simulink model "DYNctl_ver4_etud_Avec_AsservissementNONfonctionnel"  (R2021b)
settings: Solver=ode45  StartTime=0.0  StopTime=tfin  FixedStep=0.001  RelTol=1e-09  EnableMultiTasking=on
values from neighbouring files (symbols this model uses):
  A = num_pos_sph(3)    [Compensateur.m]    (also in matrice_L.m = sym(zeros(13, 13)))
  ae0 = 0.000013398315537 * 1.0e+5    (= 1.3398315537)    [bancEssaiConstantes.m]
  ae1 = 0.003556457401249 * 1.0e+5    (= 355.645740125)    [bancEssaiConstantes.m]
  ae2 = 0.018168930792891 * 1.0e+5    (= 1816.89307929)    [bancEssaiConstantes.m]
  ae3 = 7.043847497815494 * 1.0e+5    (= 704384.749782)    [bancEssaiConstantes.m]
  as0 = 0.0609    [bancEssaiConstantes.m]
  as1 = 18.1233    [bancEssaiConstantes.m]
  as2 = 3.1142e+03    (= 3114.2)    [bancEssaiConstantes.m]
  as3 = -2.3281e+05    (= -232810)    [bancEssaiConstantes.m]
  Axeq = 0    [run_bancessai.m]
  Ayeq = 0    [run_bancessai.m]
  B = [B1 ... (first row only)    [matrice_L.m]
  be1 = 13.029359254409743    (= 13.0293592544)    [bancEssaiConstantes.m]
  C = [Tdef C3 C3 C3 C2 ... (first row only)    [matrice_L.m]
  D = [sum(distance);sum(distance.*voltage)]    [Capteur.m]    (also in matrice_L.m = [0])
  g = 9.81    [bancEssaiConstantes.m]    (also in courant_voltage.m; matrice_L.m; projet.m; trajectoire.m = sqrt(1+(yd).^2))
  Jy = Jx    (= 0.001169)    [bancEssaiConstantes.m]    (also in courant_voltage.m = 0.001347; matrice_L.m = 0.001347)
  Kp_pos_sph = (wn_pos_sph^2)/A_pos_sph    [Compensateur_position_sphere.m]
  Kv_pos_sph = (2*zeta_pos_sph*wn_pos_sph)/A_pos_sph    [Compensateur_position_sphere.m]
  LA = LL    (= 0.115)    [bancEssaiConstantes.m]
  LB = LL    (= 0.115)    [bancEssaiConstantes.m]
  LC = LL    (= 0.115)    [bancEssaiConstantes.m]
  mS = 0.0080    (= 0.008)    [bancEssaiConstantes.m]
  mtot = mP + sig*mS    [bancEssaiConstantes.m]
  Px_eq_simu = double(Px_eq)    [matrice_L.m]
  Py_eq_simu = double(Py_eq)    [matrice_L.m]
  Pzeq = .015    (= 0.015)    [run_bancessai.m]
  RA = RR    (= 3.6)    [bancEssaiConstantes.m]
  RB = RR    (= 3.6)    [bancEssaiConstantes.m]
  RC = RR    (= 3.6)    [bancEssaiConstantes.m]
  TABC_inv = inv(TABC)    [bancEssaiConstantes.m]
  TDEF_inv = inv(TDEF)    [bancEssaiConstantes.m]
  Uinv = inv(U)    [matrice_L.m]
  Va_eq_simu = double(Va_eq)    [courant_voltage.m]
  Vb_eq_simu = double(Vb_eq)    [courant_voltage.m]
  Vc_eq_simu = double(Vc_eq)    [courant_voltage.m]
  Vmax = 22.0    (= 22)    [bancEssaiConstantes.m]
  XB = -rABC*sind(30)    [bancEssaiConstantes.m]    (also in courant_voltage.m = - XA*sind(30); matrice_L.m = -XA*sind(30); projet.m = XA*sind(30))
  XC = -rABC*sind(30)    [bancEssaiConstantes.m]    (also in courant_voltage.m = - XA*sind(30); matrice_L.m = -XA*sind(30); projet.m = XA*sind(30))
  YB = +rABC*cosd(30)    [bancEssaiConstantes.m]    (also in courant_voltage.m = XA*cosd(30); matrice_L.m = XA*cosd(30))
  YC = -rABC*cosd(30)    [bancEssaiConstantes.m]    (also in courant_voltage.m = -XA*cosd(30); matrice_L.m = -XA*cosd(30))
undefined symbols (not defined in the file or in its folder): A_phi, A_s, A_theta, A_z, B_phi, B_sx, B_sy, B_theta, B_z, C_dec, C_s, D_dec, D_s, den_hpc2, den_ip, num_hpc2, num_ip, Tdeft, Tdeft2, U_U_simu
(part 1 of 2)
settings Model: Creator=delafontaine  LastModifiedBy=fadd
settings SolverCC: AlgebraicLoopSolver=LineSearch
settings DataIOCC: LimitDataPoints=on  SaveFormat=Array  SignalLoggingSaveFormat=ModelDataLogs  ReturnWorkspaceOutputs=off
settings OptimizationCC: LifeSpan=inf
settings DebuggingCC: UnderspecifiedInitializationDetection=Classic  MergeDetectMultiDrivingBlocksExec=none  MultiTaskDSMMsg=warning  MultiTaskCondExecSysMsg=none  SFUnexpectedBacktrackingDiag=warning  SFNoUnconditionalDefaultTransitionDiag=warning  SFExecutionAtInitializationDiag=none  SFMachineParentedDataDiag=warning  ArithmeticOperatorsInVariantConditions=warning
settings HardwareCC: ProdBitPerPointer=32  ProdBitPerSizeT=32  ProdBitPerPtrDiffT=32  ProdLargestAtomicFloat=None  ProdIntDivRoundTo=Undefined  ProdEndianess=Unspecified  ProdWordSize=32  ProdHWDeviceType=32-bit Generic
settings ModelReferenceCC: PropagateSignalLabelsOutOfModel=off
settings SFSimCC: SimUseLocalCustomCode=off  CustomCodeUndefinedFunction=UseInterfaceOnly
settings RTWCC: RTWUseLocalCustomCode=off
settings CodeAppCC: StateflowObjectComments=on
settings GRTTargetCC: TargetLangStandard=C89/C90 (ANSI)
settings ConfigComp: CovMetricSettings=dw  CovSaveCumulativeToWorkspaceVar=on  CovSaveSingleToWorkspaceVar=on  CovExternalEMLEnable=off  CovSFcnEnable=off

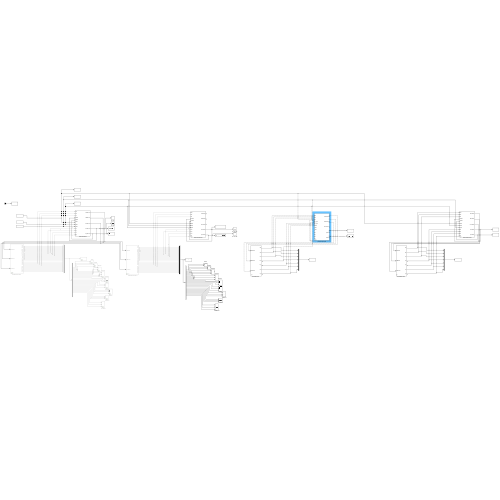
[thumbnail: Simulink's stored preview of the top-level diagram]
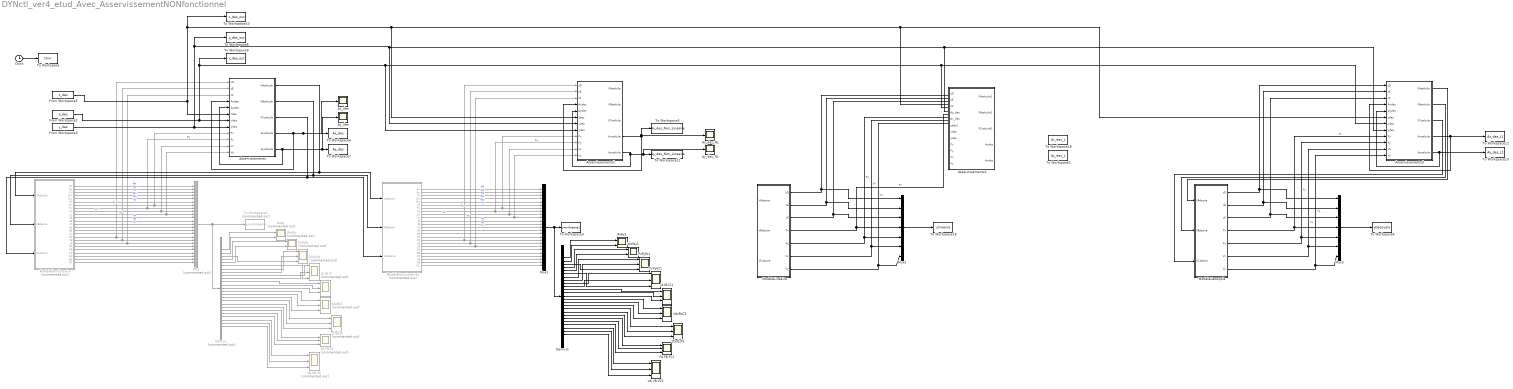
== system DYNctl_ver4_etud_Avec_AsservissementNONfonctionnel ==
  Asservissements : Subsystem
      mask help: Simulink:masks:GenSFuncDesc_MD
      mask Help: eval('feval(''rtwprivate'',''rtwhelpview'',''rtw_sfcn_block'')');
  Asservissements1 : Subsystem
      mask help: Simulink:masks:GenSFuncDesc_MD
      mask Help: eval('feval(''rtwprivate'',''rtwhelpview'',''rtw_sfcn_block'')');
  Asservissements2 : Subsystem
      mask help: Simulink:masks:GenSFuncDesc_MD
      mask Help: eval('feval(''rtwprivate'',''rtwhelpview'',''rtw_sfcn_block'')');
  Asservissements3 : Subsystem
      mask help: Simulink:masks:GenSFuncDesc_MD
      mask Help: eval('feval(''rtwprivate'',''rtwhelpview'',''rtw_sfcn_block'')');
  AxAy : Scope  Commented=on  NumInputPorts=2
  AxAy1 : Scope  NumInputPorts=2
  Ax_des : Scope
  Ax_des_NL : Scope
  Ay_des : Scope
  Ay_des_NL : Scope
  Clock : Clock
  Demux : Demux  Commented=on  Outputs=25
  Demux1 : Demux  Outputs=25
  FA FB FC : Scope  Commented=on  NumInputPorts=3
  FA FB FC1 : Scope  NumInputPorts=3
  From Workspace2 : FromWorkspace  VariableName=x_des  Interpolate=off  OutputAfterFinalValue=Holding final value
  From Workspace3 : FromWorkspace  VariableName=y_des  Interpolate=off  OutputAfterFinalValue=Holding final value
  From Workspace5 : FromWorkspace  VariableName=z_des  Interpolate=off  OutputAfterFinalValue=Holding final value
  IA IB IC : Scope  Commented=on  NumInputPorts=3
  IA IB IC1 : Scope  NumInputPorts=3
  ModeleDecouple : Subsystem
      mask help: Simulink:masks:GenSFuncDesc_MD
      mask Help: eval('feval(''rtwprivate'',''rtwhelpview'',''rtw_sfcn_block'')');
  ModeleLinéaire : Subsystem
      mask help: Simulink:masks:GenSFuncDesc_MD
      mask Help: eval('feval(''rtwprivate'',''rtwhelpview'',''rtw_sfcn_block'')');
  ModeleNonLineaire : Subsystem  Commented=on
      mask help: Simulink:masks:GenSFuncDesc_MD
      mask Help: eval('feval(''rtwprivate'',''rtwhelpview'',''rtw_sfcn_block'')');
  ModeleNonLineaire1 : Subsystem  Commented=on
      mask help: Simulink:masks:GenSFuncDesc_MD
      mask Help: eval('feval(''rtwprivate'',''rtwhelpview'',''rtw_sfcn_block'')');
  Mux : Mux  Commented=on  Inputs=25
  Mux1 : Mux  Inputs=25
  Mux2 : Mux  Inputs=7
  Mux3 : Mux  Inputs=7
  PxPyPz : Scope  Commented=on  NumInputPorts=3
  PxPyPz1 : Scope  NumInputPorts=3
  To Workspace : ToWorkspace  VariableName=tsim  SampleTime=-1
  To Workspace1 : ToWorkspace  Commented=on  VariableName=ynonlineaire  SampleTime=-1
  To Workspace10 : ToWorkspace  VariableName=z_des_out  SampleTime=-1
  To Workspace11 : ToWorkspace  VariableName=Ay_des_Non_Lineaire  SampleTime=-1
  To Workspace12 : ToWorkspace  VariableName=Ax_des_L1  SampleTime=-1
  To Workspace13 : ToWorkspace  VariableName=Ay_des_L1  SampleTime=-1
  To Workspace16 : ToWorkspace  VariableName=ylineaire  SampleTime=-1
  To Workspace18 : ToWorkspace  VariableName=Ax_des_L  SampleTime=-1
  To Workspace2 : ToWorkspace  VariableName=Ay_des_L  SampleTime=-1
  To Workspace3 : ToWorkspace  VariableName=ynonlineaire1  SampleTime=-1
  To Workspace4 : ToWorkspace  VariableName=yDecouple  SampleTime=-1
  To Workspace5 : ToWorkspace  VariableName=Ax_des_Non_Lineaire  SampleTime=-1
  To Workspace6 : ToWorkspace  VariableName=Ax_des  SampleTime=-1
  To Workspace7 : ToWorkspace  VariableName=Ay_des  SampleTime=-1
  To Workspace8 : ToWorkspace  VariableName=y_des_out  SampleTime=-1
  To Workspace9 : ToWorkspace  VariableName=x_des_out  SampleTime=-1
  VA VB VC : Scope  Commented=on  NumInputPorts=3
  VA VB VC1 : Scope  NumInputPorts=3
  VxVyVz : Scope  Commented=on  NumInputPorts=3
  VxVyVz1 : Scope  NumInputPorts=3
  WxWy : Scope  Commented=on  NumInputPorts=2
  WxWy1 : Scope  NumInputPorts=2
  zAzBzC : Scope  Commented=on  NumInputPorts=3
  zAzBzC1 : Scope  NumInputPorts=3
  zDzEzF : Scope  Commented=on  NumInputPorts=3
  zDzEzF1 : Scope  NumInputPorts=3
  wires:
  Mux/1 -> To Workspace1/1, Demux/1
  Clock/1 -> To Workspace/1
  ModeleNonLineaire/1(Ax) -> Mux/1  "Ax"
  ModeleNonLineaire/2(Ay) -> Mux/2  "Ay"
  ModeleNonLineaire/3(Pz) -> Mux/3  "Pz"
  ModeleNonLineaire/4(Wx) -> Mux/4  "Wx"
  ModeleNonLineaire/5(Wy) -> Mux/5  "Wy"
  ModeleNonLineaire/6(Vz) -> Mux/6  "Vz"
  ModeleNonLineaire/7(Px) -> Asservissements/9(Px), Mux/7  "Px"
  ModeleNonLineaire/8(Py) -> Asservissements/10(Py), Mux/8  "Py"
  ModeleNonLineaire/9(Vx) -> Asservissements/11(Vx), Mux/9  "Vx"
  ModeleNonLineaire/10(Vy) -> Asservissements/12(Vy), Mux/10  "Vy"
  ModeleNonLineaire/11(IA) -> Mux/11  "IA"
  ModeleNonLineaire/12(IB) -> Mux/12  "IB"
  ModeleNonLineaire/13(IC) -> Mux/13  "IC"
  ModeleNonLineaire/20(FA) -> Mux/20
  ModeleNonLineaire/21(FB) -> Mux/21
  ModeleNonLineaire/22(FC) -> Mux/22
  ModeleNonLineaire/23(VA) -> Mux/23
  ModeleNonLineaire/24(VB) -> Mux/24
  ModeleNonLineaire/25(VC) -> Mux/25
  ModeleNonLineaire/17(zD) -> Asservissements/1(zD), Mux/17
  ModeleNonLineaire/18(zE) -> Asservissements/2(zE), Mux/18
  ModeleNonLineaire/19(zF) -> Asservissements/3(zF), Mux/19
  ModeleNonLineaire/14(zA) -> Mux/14
  ModeleNonLineaire/15(zB) -> Mux/15
  ModeleNonLineaire/16(zC) -> Mux/16
  Asservissements/4(Axcalcule) -> Asservissements/4(Axdes), Ax_des/1, To Workspace6/1
  Asservissements/5(Aycalcule) -> Asservissements/5(Aydes), Ay_des/1, To Workspace7/1
  Asservissements/1(VAcalcule) -> ModeleNonLineaire1/1(VAdesire), ModeleNonLineaire/1(VAdesire)
  Asservissements/2(VBcalcule) -> ModeleNonLineaire1/2(VBdesire), ModeleNonLineaire/2(VBdesire)
  Asservissements/3(VCcalcule) -> ModeleNonLineaire1/3(VCdesire), ModeleNonLineaire/3(VCdesire)
  ModeleNonLineaire1/21(FB) -> Mux1/21
  ModeleNonLineaire1/16(zC) -> Mux1/16
  ModeleNonLineaire1/15(zB) -> Mux1/15
  ModeleNonLineaire1/5(Wy) -> Mux1/5  "Wy"
  ModeleNonLineaire1/23(VA) -> Mux1/23
  ModeleNonLineaire1/10(Vy) -> Asservissements1/12(Vy), Mux1/10  "Vy"
  ModeleNonLineaire1/25(VC) -> Mux1/25
  ModeleNonLineaire1/22(FC) -> Mux1/22
  ModeleNonLineaire1/20(FA) -> Mux1/20
  ModeleNonLineaire1/17(zD) -> Asservissements1/1(zD), Mux1/17
  ModeleNonLineaire1/12(IB) -> Mux1/12  "IB"
  ModeleNonLineaire1/1(Ax) -> Mux1/1  "Ax"
  ModeleNonLineaire1/13(IC) -> Mux1/13  "IC"
  ModeleNonLineaire1/3(Pz) -> Mux1/3  "Pz"
  ModeleNonLineaire1/7(Px) -> Asservissements1/9(Px), Mux1/7  "Px"
  ModeleNonLineaire1/8(Py) -> Asservissements1/10(Py), Mux1/8  "Py"
  ModeleNonLineaire1/19(zF) -> Asservissements1/3(zF), Mux1/19
  ModeleNonLineaire1/18(zE) -> Asservissements1/2(zE), Mux1/18
  ModeleNonLineaire1/9(Vx) -> Asservissements1/11(Vx), Mux1/9  "Vx"
  ModeleNonLineaire1/2(Ay) -> Mux1/2  "Ay"
  ModeleNonLineaire1/6(Vz) -> Mux1/6  "Vz"
  ModeleNonLineaire1/24(VB) -> Mux1/24
  ModeleNonLineaire1/11(IA) -> Mux1/11  "IA"
  Asservissements1/5(Aycalcule) -> Asservissements1/5(Aydes), Ay_des_NL/1, To Workspace11/1
  ModeleNonLineaire1/4(Wx) -> Mux1/4  "Wx"
  ModeleNonLineaire1/14(zA) -> Mux1/14
  ? -> ModeleLinéaire/3(VCdesire)
  ModeleLinéaire/5(Py) -> Mux2/5  "Py"
  ModeleLinéaire/1(zD) -> Mux2/1
  Mux2/1 -> To Workspace16/1
  ? -> To Workspace18/1
  ModeleLinéaire/6(Vx) -> Mux2/6  "Vx"
  ModeleLinéaire/4(Px) -> Mux2/4  "Px"
  ? -> ModeleLinéaire/1(VAdesire)
  ModeleLinéaire/3(zF) -> Mux2/3
  ? -> ModeleLinéaire/2(VBdesire)
  ModeleLinéaire/2(zE) -> Mux2/2
  ? -> To Workspace2/1
  ModeleLinéaire/7(Vy) -> Mux2/7  "Vy"
  Asservissements1/4(Axcalcule) -> Ax_des_NL/1, To Workspace5/1, Asservissements1/4(Axdes)
  Demux/1 -> AxAy/1
  Demux/3 -> PxPyPz/3
  Demux/4 -> WxWy/1
  Demux/5 -> WxWy/2
  Demux/6 -> VxVyVz/3
  Demux/7 -> PxPyPz/1
  Demux/8 -> PxPyPz/2
  Demux/9 -> VxVyVz/1
  Demux/10 -> VxVyVz/2
  Demux/11 -> IA IB IC/1
  Demux/12 -> IA IB IC/2
  Demux/13 -> IA IB IC/3
  Demux/14 -> zAzBzC/1
  Demux/15 -> zAzBzC/2
  Demux/16 -> zAzBzC/3
  Demux/17 -> zDzEzF/1
  Demux/18 -> zDzEzF/2
  Demux/19 -> zDzEzF/3
  Demux/20 -> FA FB FC/1
  Demux/21 -> FA FB FC/2
  Demux/22 -> FA FB FC/3
  Demux/23 -> VA VB VC/1
  Demux/24 -> VA VB VC/2
  Demux/25 -> VA VB VC/3
  Demux/2 -> AxAy/2
  Demux1/25 -> VA VB VC1/3
  Demux1/9 -> VxVyVz1/1
  Demux1/21 -> FA FB FC1/2
  Demux1/14 -> zAzBzC1/1
  Demux1/10 -> VxVyVz1/2
  Demux1/19 -> zDzEzF1/3
  Demux1/4 -> WxWy1/1
  Demux1/16 -> zAzBzC1/3
  Demux1/20 -> FA FB FC1/1
  Demux1/13 -> IA IB IC1/3
  Demux1/1 -> AxAy1/1
  Demux1/24 -> VA VB VC1/2
  Demux1/22 -> FA FB FC1/3
  Demux1/18 -> zDzEzF1/2
  Demux1/6 -> VxVyVz1/3
  Demux1/3 -> PxPyPz1/3
  Demux1/8 -> PxPyPz1/2
  Demux1/17 -> zDzEzF1/1
  Demux1/2 -> AxAy1/2
  Demux1/5 -> WxWy1/2
  Demux1/7 -> PxPyPz1/1
  Demux1/11 -> IA IB IC1/1
  Demux1/12 -> IA IB IC1/2
  Demux1/15 -> zAzBzC1/2
  Mux1/1 -> Demux1/1, To Workspace3/1
  Demux1/23 -> VA VB VC1/1
  Asservissements3/2(VBcalcule) -> ModeleDecouple/2(VBdesire)
  ModeleDecouple/4(Px) -> Asservissements3/9(Px), Mux3/4  "Px"
  ModeleDecouple/7(Vy) -> Asservissements3/12(Vy), Mux3/7  "Vy"
  From Workspace2/1 -> Asservissements/7(xdes), Asservissements3/7(xdes), Asservissements1/8(ydes), To Workspace9/1
  Asservissements3/4(Axcalcule) -> Asservissements3/4(Axdes), To Workspace12/1
  ModeleDecouple/2(zE) -> Asservissements3/2(zE), Mux3/2
  ModeleDecouple/6(Vx) -> Asservissements3/11(Vx), Mux3/6  "Vx"
  ModeleDecouple/3(zF) -> Asservissements3/3(zF), Mux3/3
  From Workspace5/1 -> Asservissements/6(zdes), Asservissements3/6(zdes), Asservissements1/6(zdes), To Workspace10/1
  Asservissements3/1(VAcalcule) -> ModeleDecouple/1(VAdesire)
  Asservissements3/5(Aycalcule) -> Asservissements3/5(Aydes), To Workspace13/1
  Mux3/1 -> To Workspace4/1
  Asservissements3/3(VCcalcule) -> ModeleDecouple/3(VCdesire)
  From Workspace3/1 -> Asservissements/8(ydes), Asservissements3/8(ydes), Asservissements1/7(xdes), To Workspace8/1
  ModeleDecouple/5(Py) -> Asservissements3/10(Py), Mux3/5  "Py"
  ModeleDecouple/1(zD) -> Asservissements3/1(zD), Mux3/1

== system DYNctl_ver4_etud_Avec_AsservissementNONfonctionnel/Asservissements ==
  zD : Inport
  zE : Inport  Port=2
  zF : Inport  Port=3
  Axdes : Inport  Port=4
  Aydes : Inport  Port=5
  zdes : Inport  Port=6
  xdes : Inport  Port=7
  ydes : Inport  Port=8
  Px : Inport  Port=9
  Py : Inport  Port=10
  Vx : Inport  Port=11
  Vy : Inport  Port=12
  Asservissements_sfcn : S-Function  FunctionName=Asservissements_sf  SFunctionModules=""  SFunctionDeploymentMode=off  EnableBusSupport=off  mask{rtw_sf_name=Asservissements_sf, showVar=off}
      mask prompts: rtw_sf_name "Simulink:masks:GenSFuncName_MP"; showVar "Simulink:masks:GenSFuncShowModuleList_MP"
      mask help: Simulink:masks:GenSFuncDesc_MD
      mask init:
      | displist = '';
      | if ~strcmp(get_param(gcb, 'FunctionName'), rtw_sf_name);
      |   set_param(gcb, 'FunctionName', rtw_sf_name);
      | end
      | % Check if we are generating code
      | rtw_mode = false;
      | if strcmpi(get_param(bdroot(gcb),'SimulationStatus'),'Initializing')
      | 	rtw_mode = strcmpi(get_param(bdroot(gcb),'BuildingRTWCode'),'on') && ...
      | 		~strcmpi(get_param(bdroot(gcb),'TargetStyle'),'SimulationTarget');
      | end
      | if showVar || rtw_mode
      | 	if exist('rtwsfunc') == 2 | exist('rtwsfunc') == 6
      | 		tmplist = rtwsfunc(rtw_sf_name,gcb);
      | 		tmplist = DAStudio.message('Simulink:masks:GenSFuncListOfModules_IC', tmplist);
      | 	elseif showVar
      | 		tmplist1 = DAStudio.message('Simulink:masks:GenSFuncListOfModules_IC', '');
      |         tmplist2 = DAStudio.message('Simulink:masks:GenSFuncNotLicensed_IC');
      |         tmplist = [tmplist1 tmplist2];
      |  	end
      | end
      | if showVar
      |   displist = tmplist;
      | end
      settings: CopyFcn=|
      | if ~strcmp(get_param(gcb,'Linkstatus'),'none') && ...
      | ~strcmp(get_param(gcb,'Linkstatus'),'implicit')
      |   set_param(gcb,'LinkStatus','none');
      | end
      mask Help: eval('feval(''rtwprivate'',''rtwhelpview'',''rtw_sfcn_block'')');
      mask Display:
      | port_label('input',1,'zD');
      | port_label('input',2,'zE');
      | port_label('input',3,'zF');
      | port_label('input',4,'Axdes');
      | port_label('input',5,'Aydes');
      | port_label('input',6,'zdes');
      | port_label('input',7,'xdes');
      | port_label('input',8,'ydes');
      | port_label('input',9,'Px');
      | port_label('input',10,'Py');
      | port_label('input',11,'Vx');
      | port_label('input',12,'Vy');
      | port_label('output',1,'VAcalcule');
      | port_label('output',2,'VBcalcule');
      | port_label('output',3,'VCcalcule');
      | port_label('output',4,'Axcalcule');
      | port_label('output',5,'Aycalcule');
  __InputSSForSFun__ : Subsystem
  __OutputSSForSFun__ : Subsystem
  VAcalcule : Outport
  VBcalcule : Outport  Port=2
  VCcalcule : Outport  Port=3
  Axcalcule : Outport  Port=4
  Aycalcule : Outport  Port=5
  wires:
  zD/1 -> __InputSSForSFun__/1(zD)
  zE/1 -> __InputSSForSFun__/2(zE)
  zF/1 -> __InputSSForSFun__/3(zF)
  Axdes/1 -> __InputSSForSFun__/4(Axdes)
  Aydes/1 -> __InputSSForSFun__/5(Aydes)
  zdes/1 -> __InputSSForSFun__/6(zdes)
  xdes/1 -> __InputSSForSFun__/7(xdes)
  Px/1 -> __InputSSForSFun__/9(Px)
  Py/1 -> __InputSSForSFun__/10(Py)
  Vx/1 -> __InputSSForSFun__/11(Vx)
  Vy/1 -> __InputSSForSFun__/12(Vy)
  __InputSSForSFun__/1(__UniqueOutportName__1__) -> Asservissements_sfcn/1
  __InputSSForSFun__/2(__UniqueOutportName__2__) -> Asservissements_sfcn/2
  __InputSSForSFun__/3(__UniqueOutportName__3__) -> Asservissements_sfcn/3
  __InputSSForSFun__/4(__UniqueOutportName__4__) -> Asservissements_sfcn/4
  __InputSSForSFun__/5(__UniqueOutportName__5__) -> Asservissements_sfcn/5
  __InputSSForSFun__/6(__UniqueOutportName__6__) -> Asservissements_sfcn/6
  __InputSSForSFun__/7(__UniqueOutportName__7__) -> Asservissements_sfcn/7
  __InputSSForSFun__/8(__UniqueOutportName__8__) -> Asservissements_sfcn/8
  __InputSSForSFun__/9(__UniqueOutportName__9__) -> Asservissements_sfcn/9
  __InputSSForSFun__/10(__UniqueOutportName__10__) -> Asservissements_sfcn/10
  __InputSSForSFun__/11(__UniqueOutportName__11__) -> Asservissements_sfcn/11
  __InputSSForSFun__/12(__UniqueOutportName__12__) -> Asservissements_sfcn/12
  Asservissements_sfcn/1 -> __OutputSSForSFun__/1(__UniqueInportName__1__)
  Asservissements_sfcn/2 -> __OutputSSForSFun__/2(__UniqueInportName__2__)
  Asservissements_sfcn/3 -> __OutputSSForSFun__/3(__UniqueInportName__3__)
  Asservissements_sfcn/4 -> __OutputSSForSFun__/4(__UniqueInportName__4__)
  Asservissements_sfcn/5 -> __OutputSSForSFun__/5(__UniqueInportName__5__)
  __OutputSSForSFun__/1(VAcalcule) -> VAcalcule/1
  __OutputSSForSFun__/2(VBcalcule) -> VBcalcule/1
  __OutputSSForSFun__/3(VCcalcule) -> VCcalcule/1
  __OutputSSForSFun__/4(Axcalcule) -> Axcalcule/1
  __OutputSSForSFun__/5(Aycalcule) -> Aycalcule/1
  ydes/1 -> __InputSSForSFun__/8(ydes)

== system DYNctl_ver4_etud_Avec_AsservissementNONfonctionnel/Asservissements1 ==
  zD : Inport
  zE : Inport  Port=2
  zF : Inport  Port=3
  Axdes : Inport  Port=4
  Aydes : Inport  Port=5
  zdes : Inport  Port=6
  xdes : Inport  Port=7
  ydes : Inport  Port=8
  Px : Inport  Port=9
  Py : Inport  Port=10
  Vx : Inport  Port=11
  Vy : Inport  Port=12
  Asservissements_sfcn : S-Function  FunctionName=Asservissements_sf  SFunctionModules=""  SFunctionDeploymentMode=off  EnableBusSupport=off  mask{rtw_sf_name=Asservissements_sf, showVar=off}
      mask prompts: rtw_sf_name "Simulink:masks:GenSFuncName_MP"; showVar "Simulink:masks:GenSFuncShowModuleList_MP"
      mask help: Simulink:masks:GenSFuncDesc_MD
      mask init: same as DYNctl_ver4_etud_Avec_AsservissementNONfonctionnel/Asservissements/Asservissements_sfcn
      settings: CopyFcn=|
      | if ~strcmp(get_param(gcb,'Linkstatus'),'none') && ...
      | ~strcmp(get_param(gcb,'Linkstatus'),'implicit')
      |   set_param(gcb,'LinkStatus','none');
      | end
      mask Help: eval('feval(''rtwprivate'',''rtwhelpview'',''rtw_sfcn_block'')');
      mask Display:
      | port_label('input',1,'zD');
      | port_label('input',2,'zE');
      | port_label('input',3,'zF');
      | port_label('input',4,'Axdes');
      | port_label('input',5,'Aydes');
      | port_label('input',6,'zdes');
      | port_label('input',7,'xdes');
      | port_label('input',8,'ydes');
      | port_label('input',9,'Px');
      | port_label('input',10,'Py');
      | port_label('input',11,'Vx');
      | port_label('input',12,'Vy');
      | port_label('output',1,'VAcalcule');
      | port_label('output',2,'VBcalcule');
      | port_label('output',3,'VCcalcule');
      | port_label('output',4,'Axcalcule');
      | port_label('output',5,'Aycalcule');
  __InputSSForSFun__ : Subsystem
  __OutputSSForSFun__ : Subsystem
  VAcalcule : Outport
  VBcalcule : Outport  Port=2
  VCcalcule : Outport  Port=3
  Axcalcule : Outport  Port=4
  Aycalcule : Outport  Port=5
  wires:
  __InputSSForSFun__/1(__UniqueOutportName__1__) -> Asservissements_sfcn/1
  __InputSSForSFun__/2(__UniqueOutportName__2__) -> Asservissements_sfcn/2
  __InputSSForSFun__/3(__UniqueOutportName__3__) -> Asservissements_sfcn/3
  __InputSSForSFun__/4(__UniqueOutportName__4__) -> Asservissements_sfcn/4
  __InputSSForSFun__/5(__UniqueOutportName__5__) -> Asservissements_sfcn/5
  __InputSSForSFun__/6(__UniqueOutportName__6__) -> Asservissements_sfcn/6
  __InputSSForSFun__/7(__UniqueOutportName__7__) -> Asservissements_sfcn/7
  __InputSSForSFun__/8(__UniqueOutportName__8__) -> Asservissements_sfcn/8
  __InputSSForSFun__/9(__UniqueOutportName__9__) -> Asservissements_sfcn/9
  __InputSSForSFun__/10(__UniqueOutportName__10__) -> Asservissements_sfcn/10
  __InputSSForSFun__/11(__UniqueOutportName__11__) -> Asservissements_sfcn/11
  __InputSSForSFun__/12(__UniqueOutportName__12__) -> Asservissements_sfcn/12
  Asservissements_sfcn/1 -> __OutputSSForSFun__/1(__UniqueInportName__1__)
  Asservissements_sfcn/2 -> __OutputSSForSFun__/2(__UniqueInportName__2__)
  Asservissements_sfcn/3 -> __OutputSSForSFun__/3(__UniqueInportName__3__)
  Asservissements_sfcn/4 -> __OutputSSForSFun__/4(__UniqueInportName__4__)
  Asservissements_sfcn/5 -> __OutputSSForSFun__/5(__UniqueInportName__5__)
  __OutputSSForSFun__/1(VAcalcule) -> VAcalcule/1
  __OutputSSForSFun__/2(VBcalcule) -> VBcalcule/1
  __OutputSSForSFun__/3(VCcalcule) -> VCcalcule/1
  __OutputSSForSFun__/4(Axcalcule) -> Axcalcule/1
  __OutputSSForSFun__/5(Aycalcule) -> Aycalcule/1
  Vy/1 -> __InputSSForSFun__/12(Vy)
  Axdes/1 -> __InputSSForSFun__/4(Axdes)
  zE/1 -> __InputSSForSFun__/2(zE)
  Vx/1 -> __InputSSForSFun__/11(Vx)
  zD/1 -> __InputSSForSFun__/1(zD)
  Aydes/1 -> __InputSSForSFun__/5(Aydes)
  zF/1 -> __InputSSForSFun__/3(zF)
  Px/1 -> __InputSSForSFun__/9(Px)
  Py/1 -> __InputSSForSFun__/10(Py)
  ydes/1 -> __InputSSForSFun__/8(ydes)
  xdes/1 -> __InputSSForSFun__/7(xdes)
  zdes/1 -> __InputSSForSFun__/6(zdes)

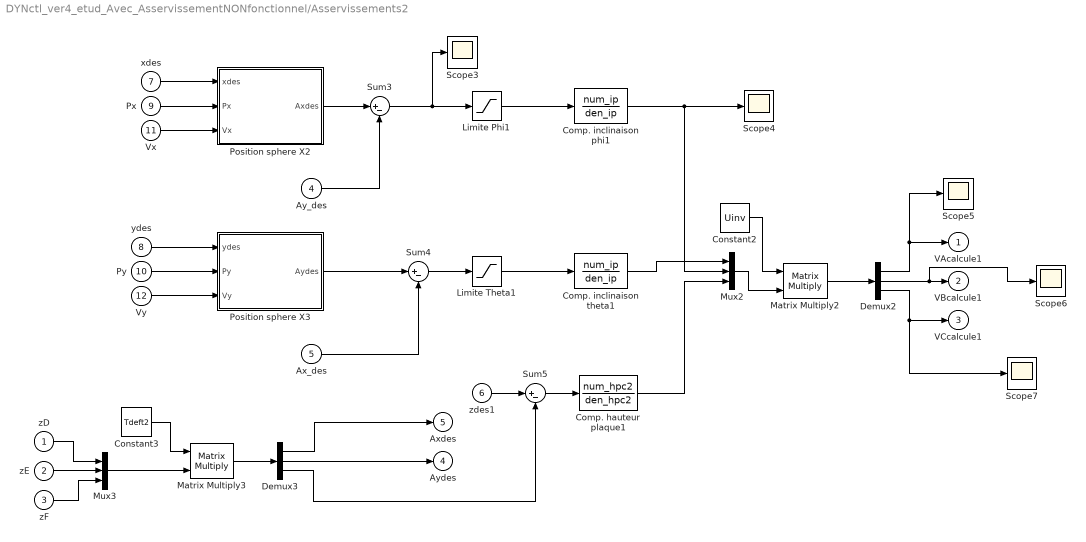
== system DYNctl_ver4_etud_Avec_AsservissementNONfonctionnel/Asservissements2 ==
  zD : Inport
  zE : Inport  Port=2
  zF : Inport  Port=3
  Ay_des : Inport  Port=4
  Ax_des : Inport  Port=5
  zdes1 : Inport  Port=6
  xdes : Inport  Port=7
  ydes : Inport  Port=8
  Px : Inport  Port=9
  Py : Inport  Port=10
  Vx : Inport  Port=11
  Vy : Inport  Port=12
  Comp. hauteur plaque1 : TransferFcn  Numerator=num_hpc2  Denominator=den_hpc2
  Comp. inclinaison phi1 : TransferFcn  Numerator=num_ip  Denominator=den_ip
  Comp. inclinaison theta1 : TransferFcn  Numerator=num_ip  Denominator=den_ip
  Constant2 : Constant  Value=Uinv
  Constant3 : Constant  Value=Tdeft2
  Demux2 : Demux  Outputs=3
  Demux3 : Demux  Outputs=3
  Limite Phi1 : Saturate  UpperLimit=5  LowerLimit=5
  Limite Theta1 : Saturate  UpperLimit=5  LowerLimit=5
  Matrix Multiply2 : Product  Multiplication=Matrix(*)
  Matrix Multiply3 : Product  Multiplication=Matrix(*)
  Mux2 : Mux  Inputs=3
  Mux3 : Mux  Inputs=3
  Position sphere X2 : Subsystem
  Position sphere X3 : Subsystem
  Scope{3..7} (5 alike) : Scope
  Sum3 : Sum  Inputs=|+-
  Sum4 : Sum  Inputs=|+-
  Sum5 : Sum  Inputs=|+-
  VAcalcule1 : Outport  VectorParamsAs1DForOutWhenUnconnected=off
  VBcalcule1 : Outport  Port=2  VectorParamsAs1DForOutWhenUnconnected=off
  VCcalcule1 : Outport  Port=3  VectorParamsAs1DForOutWhenUnconnected=off
  Aydes : Outport  Port=4  VectorParamsAs1DForOutWhenUnconnected=off
  Axdes : Outport  Port=5  VectorParamsAs1DForOutWhenUnconnected=off
  wires:
  Comp. inclinaison theta1/1 -> Mux2/1
  Ax_des/1 -> Sum4/2
  Limite Theta1/1 -> Comp. inclinaison theta1/1
  Mux2/1 -> Matrix Multiply2/2
  Demux3/2 -> Aydes/1
  ydes/1 -> Position sphere X3/1(ydes)
  Position sphere X2/1(Axdes) -> Sum3/1
  zD/1 -> Mux3/1
  Demux2/1 -> Scope5/1, VAcalcule1/1
  zE/1 -> Mux3/2
  Position sphere X3/1(Aydes) -> Sum4/1
  Vy/1 -> Position sphere X3/3(Vy)
  Matrix Multiply2/1 -> Demux2/1
  xdes/1 -> Position sphere X2/1(xdes)
  Demux2/3 -> VCcalcule1/1, Scope7/1
  Matrix Multiply3/1 -> Demux3/1
  zF/1 -> Mux3/3
  Demux3/1 -> Axdes/1
  Vx/1 -> Position sphere X2/3(Vx)
  Py/1 -> Position sphere X3/2(Py)
  Constant2/1 -> Matrix Multiply2/1
  Demux2/2 -> Scope6/1, VBcalcule1/1
  Px/1 -> Position sphere X2/2(Px)
  Sum4/1 -> Limite Theta1/1
  Mux3/1 -> Matrix Multiply3/2
  Demux3/3 -> Sum5/2
  Sum5/1 -> Comp. hauteur plaque1/1
  Comp. inclinaison phi1/1 -> Mux2/2, Scope4/1
  Ay_des/1 -> Sum3/2
  zdes1/1 -> Sum5/1
  Limite Phi1/1 -> Comp. inclinaison phi1/1
  Constant3/1 -> Matrix Multiply3/1
  Comp. hauteur plaque1/1 -> Mux2/3
  Sum3/1 -> Scope3/1, Limite Phi1/1

== system DYNctl_ver4_etud_Avec_AsservissementNONfonctionnel/Asservissements3 ==
  zD : Inport
  zE : Inport  Port=2
  zF : Inport  Port=3
  Axdes : Inport  Port=4
  Aydes : Inport  Port=5
  zdes : Inport  Port=6
  xdes : Inport  Port=7
  ydes : Inport  Port=8
  Px : Inport  Port=9
  Py : Inport  Port=10
  Vx : Inport  Port=11
  Vy : Inport  Port=12
  Asservissements_sfcn : S-Function  FunctionName=Asservissements_sf  SFunctionModules=""  SFunctionDeploymentMode=off  EnableBusSupport=off  mask{rtw_sf_name=Asservissements_sf, showVar=off}
      mask prompts: rtw_sf_name "Simulink:masks:GenSFuncName_MP"; showVar "Simulink:masks:GenSFuncShowModuleList_MP"
      mask help: Simulink:masks:GenSFuncDesc_MD
      mask init: same as DYNctl_ver4_etud_Avec_AsservissementNONfonctionnel/Asservissements/Asservissements_sfcn
      settings: CopyFcn=|
      | if ~strcmp(get_param(gcb,'Linkstatus'),'none') && ...
      | ~strcmp(get_param(gcb,'Linkstatus'),'implicit')
      |   set_param(gcb,'LinkStatus','none');
      | end
      mask Help: eval('feval(''rtwprivate'',''rtwhelpview'',''rtw_sfcn_block'')');
      mask Display:
      | port_label('input',1,'zD');
      | port_label('input',2,'zE');
      | port_label('input',3,'zF');
      | port_label('input',4,'Axdes');
      | port_label('input',5,'Aydes');
      | port_label('input',6,'zdes');
      | port_label('input',7,'xdes');
      | port_label('input',8,'ydes');
      | port_label('input',9,'Px');
      | port_label('input',10,'Py');
      | port_label('input',11,'Vx');
      | port_label('input',12,'Vy');
      | port_label('output',1,'VAcalcule');
      | port_label('output',2,'VBcalcule');
      | port_label('output',3,'VCcalcule');
      | port_label('output',4,'Axcalcule');
      | port_label('output',5,'Aycalcule');
  __InputSSForSFun__ : Subsystem
  __OutputSSForSFun__ : Subsystem
  VAcalcule : Outport  VectorParamsAs1DForOutWhenUnconnected=off
  VBcalcule : Outport  Port=2  VectorParamsAs1DForOutWhenUnconnected=off
  VCcalcule : Outport  Port=3  VectorParamsAs1DForOutWhenUnconnected=off
  Axcalcule : Outport  Port=4  VectorParamsAs1DForOutWhenUnconnected=off
  Aycalcule : Outport  Port=5  VectorParamsAs1DForOutWhenUnconnected=off
  wires:
  __InputSSForSFun__/1(__UniqueOutportName__1__) -> Asservissements_sfcn/1
  __InputSSForSFun__/2(__UniqueOutportName__2__) -> Asservissements_sfcn/2
  __InputSSForSFun__/3(__UniqueOutportName__3__) -> Asservissements_sfcn/3
  __InputSSForSFun__/4(__UniqueOutportName__4__) -> Asservissements_sfcn/4
  __InputSSForSFun__/5(__UniqueOutportName__5__) -> Asservissements_sfcn/5
  __InputSSForSFun__/6(__UniqueOutportName__6__) -> Asservissements_sfcn/6
  __InputSSForSFun__/7(__UniqueOutportName__7__) -> Asservissements_sfcn/7
  __InputSSForSFun__/8(__UniqueOutportName__8__) -> Asservissements_sfcn/8
  __InputSSForSFun__/9(__UniqueOutportName__9__) -> Asservissements_sfcn/9
  __InputSSForSFun__/10(__UniqueOutportName__10__) -> Asservissements_sfcn/10
  __InputSSForSFun__/11(__UniqueOutportName__11__) -> Asservissements_sfcn/11
  __InputSSForSFun__/12(__UniqueOutportName__12__) -> Asservissements_sfcn/12
  __OutputSSForSFun__/1(VAcalcule) -> VAcalcule/1
  __OutputSSForSFun__/2(VBcalcule) -> VBcalcule/1
  __OutputSSForSFun__/3(VCcalcule) -> VCcalcule/1
  __OutputSSForSFun__/4(Axcalcule) -> Axcalcule/1
  __OutputSSForSFun__/5(Aycalcule) -> Aycalcule/1
  Asservissements_sfcn/4 -> __OutputSSForSFun__/4(__UniqueInportName__4__)
  Asservissements_sfcn/5 -> __OutputSSForSFun__/5(__UniqueInportName__5__)
  Asservissements_sfcn/1 -> __OutputSSForSFun__/1(__UniqueInportName__1__)
  Asservissements_sfcn/2 -> __OutputSSForSFun__/2(__UniqueInportName__2__)
  Asservissements_sfcn/3 -> __OutputSSForSFun__/3(__UniqueInportName__3__)
  Vy/1 -> __InputSSForSFun__/12(Vy)
  Axdes/1 -> __InputSSForSFun__/4(Axdes)
  zE/1 -> __InputSSForSFun__/2(zE)
  Vx/1 -> __InputSSForSFun__/11(Vx)
  zD/1 -> __InputSSForSFun__/1(zD)
  Aydes/1 -> __InputSSForSFun__/5(Aydes)
  zF/1 -> __InputSSForSFun__/3(zF)
  Px/1 -> __InputSSForSFun__/9(Px)
  Py/1 -> __InputSSForSFun__/10(Py)
  ydes/1 -> __InputSSForSFun__/8(ydes)
  xdes/1 -> __InputSSForSFun__/7(xdes)
  zdes/1 -> __InputSSForSFun__/6(zdes)

== system DYNctl_ver4_etud_Avec_AsservissementNONfonctionnel/ModeleDecouple ==
  VAdesire : Inport
  VBdesire : Inport  Port=2
  VCdesire : Inport  Port=3
  Modeledécoupler : Subsystem
  __InputSSForSFun__ : Subsystem
  __OutputSSForSFun__ : Subsystem
  zD : Outport  VectorParamsAs1DForOutWhenUnconnected=off
  zE : Outport  Port=2  VectorParamsAs1DForOutWhenUnconnected=off
  zF : Outport  Port=3  VectorParamsAs1DForOutWhenUnconnected=off
  Px : Outport  Port=4  VectorParamsAs1DForOutWhenUnconnected=off
  Py : Outport  Port=5  VectorParamsAs1DForOutWhenUnconnected=off
  Vx : Outport  Port=6  VectorParamsAs1DForOutWhenUnconnected=off
  Vy : Outport  Port=7  VectorParamsAs1DForOutWhenUnconnected=off
  wires:
  VAdesire/1 -> __InputSSForSFun__/1(VAdesire)
  VBdesire/1 -> __InputSSForSFun__/2(VBdesire)
  VCdesire/1 -> __InputSSForSFun__/3(VCdesire)
  __InputSSForSFun__/1(__UniqueOutportName__1__) -> Modeledécoupler/1(__UniqueInportName__1__)
  __InputSSForSFun__/2(__UniqueOutportName__2__) -> Modeledécoupler/2(__UniqueInportName__2__)
  __InputSSForSFun__/3(__UniqueOutportName__3__) -> Modeledécoupler/3(__UniqueInportName__3__)
  Modeledécoupler/1(dD) -> __OutputSSForSFun__/1(__UniqueInportName__17__1)
  Modeledécoupler/4(Px) -> __OutputSSForSFun__/4(__UniqueInportName__7__)
  Modeledécoupler/5(Py) -> __OutputSSForSFun__/5(__UniqueInportName__8__)
  Modeledécoupler/6(Vx) -> __OutputSSForSFun__/6(__UniqueInportName__9__)
  Modeledécoupler/7(Vy) -> __OutputSSForSFun__/7(__UniqueInportName__10__)
  Modeledécoupler/2(dE) -> __OutputSSForSFun__/2(__UniqueInportName__18__)
  Modeledécoupler/3(dF) -> __OutputSSForSFun__/3(__UniqueInportName__19__)
  __OutputSSForSFun__/7(Vy) -> Vy/1
  __OutputSSForSFun__/6(Vx) -> Vx/1
  __OutputSSForSFun__/5(Py) -> Py/1
  __OutputSSForSFun__/4(Px) -> Px/1
  __OutputSSForSFun__/3(zF1) -> zF/1
  __OutputSSForSFun__/2(zE1) -> zE/1
  __OutputSSForSFun__/1(zD1) -> zD/1

== system DYNctl_ver4_etud_Avec_AsservissementNONfonctionnel/ModeleLinéaire ==
  VAdesire : Inport
  VBdesire : Inport  Port=2
  VCdesire : Inport  Port=3
  ModeleLineaire : Subsystem
  __InputSSForSFun__ : Subsystem
  __OutputSSForSFun__ : Subsystem
  zD : Outport  VectorParamsAs1DForOutWhenUnconnected=off
  zE : Outport  Port=2  VectorParamsAs1DForOutWhenUnconnected=off
  zF : Outport  Port=3  VectorParamsAs1DForOutWhenUnconnected=off
  Px : Outport  Port=4  VectorParamsAs1DForOutWhenUnconnected=off
  Py : Outport  Port=5  VectorParamsAs1DForOutWhenUnconnected=off
  Vx : Outport  Port=6  VectorParamsAs1DForOutWhenUnconnected=off
  Vy : Outport  Port=7  VectorParamsAs1DForOutWhenUnconnected=off
  wires:
  VAdesire/1 -> __InputSSForSFun__/1(VAdesire)
  VBdesire/1 -> __InputSSForSFun__/2(VBdesire)
  VCdesire/1 -> __InputSSForSFun__/3(VCdesire)
  __InputSSForSFun__/1(__UniqueOutportName__1__) -> ModeleLineaire/1(__UniqueInportName__1__)
  __InputSSForSFun__/2(__UniqueOutportName__2__) -> ModeleLineaire/2(__UniqueInportName__2__)
  __InputSSForSFun__/3(__UniqueOutportName__3__) -> ModeleLineaire/3(__UniqueInportName__3__)
  ModeleLineaire/1(dD) -> __OutputSSForSFun__/1(__UniqueInportName__17__)
  ModeleLineaire/2(dE) -> __OutputSSForSFun__/2(__UniqueInportName__18__)
  ModeleLineaire/3(dF) -> __OutputSSForSFun__/3(__UniqueInportName__19__)
  ModeleLineaire/4(Px) -> __OutputSSForSFun__/4(__UniqueInportName__7__)
  ModeleLineaire/5(Py) -> __OutputSSForSFun__/5(__UniqueInportName__8__)
  ModeleLineaire/6(Vx) -> __OutputSSForSFun__/6(__UniqueInportName__9__)
  ModeleLineaire/7(Vy) -> __OutputSSForSFun__/7(__UniqueInportName__10__)
  __OutputSSForSFun__/1(zD) -> zD/1
  __OutputSSForSFun__/2(zE) -> zE/1
  __OutputSSForSFun__/3(zF) -> zF/1
  __OutputSSForSFun__/4(Px) -> Px/1
  __OutputSSForSFun__/5(Py) -> Py/1
  __OutputSSForSFun__/6(Vx) -> Vx/1
  __OutputSSForSFun__/7(Vy) -> Vy/1

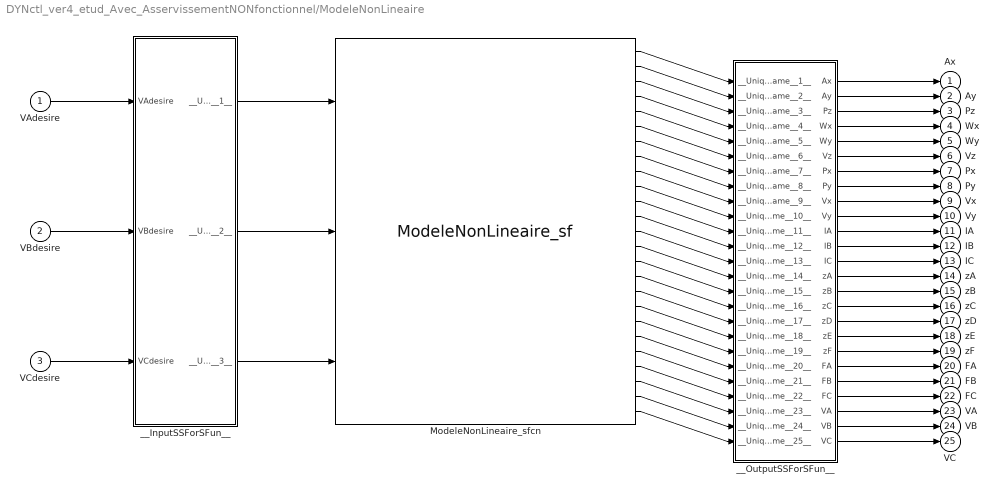
== system DYNctl_ver4_etud_Avec_AsservissementNONfonctionnel/ModeleNonLineaire ==
  VAdesire : Inport
  VBdesire : Inport  Port=2
  VCdesire : Inport  Port=3
  ModeleNonLineaire_sfcn : S-Function  FunctionName=ModeleNonLineaire_sf  SFunctionModules=""  SFunctionDeploymentMode=off  EnableBusSupport=off  mask{rtw_sf_name=ModeleNonLineaire_sf, showVar=off}
      mask prompts: rtw_sf_name "Simulink:masks:GenSFuncName_MP"; showVar "Simulink:masks:GenSFuncShowModuleList_MP"
      mask help: Simulink:masks:GenSFuncDesc_MD
      mask init: same as DYNctl_ver4_etud_Avec_AsservissementNONfonctionnel/Asservissements/Asservissements_sfcn
      settings: CopyFcn=|
      | if ~strcmp(get_param(gcb,'Linkstatus'),'none') && ...
      | ~strcmp(get_param(gcb,'Linkstatus'),'implicit')
      |   set_param(gcb,'LinkStatus','none');
      | end
      mask Help: eval('feval(''rtwprivate'',''rtwhelpview'',''rtw_sfcn_block'')');
      mask Display:
      | port_label('input',1,'VAdesire');
      | port_label('input',2,'VBdesire');
      | port_label('input',3,'VCdesire');
      | port_label('output',1,'Ax');
      | port_label('output',2,'Ay');
      | port_label('output',3,'Pz');
      | port_label('output',4,'Wx');
      | port_label('output',5,'Wy');
      | port_label('output',6,'Vz');
      | port_label('output',7,'Px');
      | port_label('output',8,'Py');
      | port_label('output',9,'Vx');
      | port_label('output',10,'Vy');
      | port_label('output',11,'IA');
      | port_label('output',12,'IB');
      | port_label('output',13,'IC');
      | port_label('output',14,'zA');
      | port_label('output',15,'zB');
      | port_label('output',16,'zC');
      | port_label('output',17,'zD');
      | port_label('output',18,'zE');
      | port_label('output',19,'zF');
      | port_label('output',20,'FA');
      | port_label('output',21,'FB');
      | port_label('output',22,'FC');
      | port_label('output',23,'VA');
      | port_label('output',24,'VB');
      | port_label('output',25,'VC');
  __InputSSForSFun__ : Subsystem
  __OutputSSForSFun__ : Subsystem
  Ax : Outport
  Ay : Outport  Port=2
  Pz : Outport  Port=3
  Wx : Outport  Port=4
  Wy : Outport  Port=5
  Vz : Outport  Port=6
  Px : Outport  Port=7
  Py : Outport  Port=8
  Vx : Outport  Port=9
  Vy : Outport  Port=10
  IA : Outport  Port=11
  IB : Outport  Port=12
  IC : Outport  Port=13
  zA : Outport  Port=14
  zB : Outport  Port=15
  zC : Outport  Port=16
  zD : Outport  Port=17
  zE : Outport  Port=18
  zF : Outport  Port=19
  FA : Outport  Port=20
  FB : Outport  Port=21
  FC : Outport  Port=22
  VA : Outport  Port=23
  VB : Outport  Port=24
  VC : Outport  Port=25
  wires:
  VAdesire/1 -> __InputSSForSFun__/1(VAdesire)
  VBdesire/1 -> __InputSSForSFun__/2(VBdesire)
  VCdesire/1 -> __InputSSForSFun__/3(VCdesire)
  __InputSSForSFun__/1(__UniqueOutportName__1__) -> ModeleNonLineaire_sfcn/1
  __InputSSForSFun__/2(__UniqueOutportName__2__) -> ModeleNonLineaire_sfcn/2
  __InputSSForSFun__/3(__UniqueOutportName__3__) -> ModeleNonLineaire_sfcn/3
  ModeleNonLineaire_sfcn/1 -> __OutputSSForSFun__/1(__UniqueInportName__1__)
  ModeleNonLineaire_sfcn/2 -> __OutputSSForSFun__/2(__UniqueInportName__2__)
  ModeleNonLineaire_sfcn/3 -> __OutputSSForSFun__/3(__UniqueInportName__3__)
  ModeleNonLineaire_sfcn/4 -> __OutputSSForSFun__/4(__UniqueInportName__4__)
  ModeleNonLineaire_sfcn/5 -> __OutputSSForSFun__/5(__UniqueInportName__5__)
  ModeleNonLineaire_sfcn/6 -> __OutputSSForSFun__/6(__UniqueInportName__6__)
  ModeleNonLineaire_sfcn/7 -> __OutputSSForSFun__/7(__UniqueInportName__7__)
  ModeleNonLineaire_sfcn/8 -> __OutputSSForSFun__/8(__UniqueInportName__8__)
  ModeleNonLineaire_sfcn/9 -> __OutputSSForSFun__/9(__UniqueInportName__9__)
  ModeleNonLineaire_sfcn/10 -> __OutputSSForSFun__/10(__UniqueInportName__10__)
  ModeleNonLineaire_sfcn/11 -> __OutputSSForSFun__/11(__UniqueInportName__11__)
  ModeleNonLineaire_sfcn/12 -> __OutputSSForSFun__/12(__UniqueInportName__12__)
  ModeleNonLineaire_sfcn/13 -> __OutputSSForSFun__/13(__UniqueInportName__13__)
  ModeleNonLineaire_sfcn/14 -> __OutputSSForSFun__/14(__UniqueInportName__14__)
  ModeleNonLineaire_sfcn/15 -> __OutputSSForSFun__/15(__UniqueInportName__15__)
  ModeleNonLineaire_sfcn/16 -> __OutputSSForSFun__/16(__UniqueInportName__16__)
  ModeleNonLineaire_sfcn/17 -> __OutputSSForSFun__/17(__UniqueInportName__17__)
  ModeleNonLineaire_sfcn/18 -> __OutputSSForSFun__/18(__UniqueInportName__18__)
  ModeleNonLineaire_sfcn/19 -> __OutputSSForSFun__/19(__UniqueInportName__19__)
  ModeleNonLineaire_sfcn/20 -> __OutputSSForSFun__/20(__UniqueInportName__20__)
  ModeleNonLineaire_sfcn/21 -> __OutputSSForSFun__/21(__UniqueInportName__21__)
  ModeleNonLineaire_sfcn/22 -> __OutputSSForSFun__/22(__UniqueInportName__22__)
  ModeleNonLineaire_sfcn/23 -> __OutputSSForSFun__/23(__UniqueInportName__23__)
  ModeleNonLineaire_sfcn/24 -> __OutputSSForSFun__/24(__UniqueInportName__24__)
  ModeleNonLineaire_sfcn/25 -> __OutputSSForSFun__/25(__UniqueInportName__25__)
  __OutputSSForSFun__/1(Ax) -> Ax/1
  __OutputSSForSFun__/2(Ay) -> Ay/1
  __OutputSSForSFun__/3(Pz) -> Pz/1
  __OutputSSForSFun__/4(Wx) -> Wx/1
  __OutputSSForSFun__/5(Wy) -> Wy/1
  __OutputSSForSFun__/6(Vz) -> Vz/1
  __OutputSSForSFun__/7(Px) -> Px/1
  __OutputSSForSFun__/8(Py) -> Py/1
  __OutputSSForSFun__/9(Vx) -> Vx/1
  __OutputSSForSFun__/10(Vy) -> Vy/1
  __OutputSSForSFun__/11(IA) -> IA/1
  __OutputSSForSFun__/12(IB) -> IB/1
  __OutputSSForSFun__/13(IC) -> IC/1
  __OutputSSForSFun__/14(zA) -> zA/1
  __OutputSSForSFun__/15(zB) -> zB/1
  __OutputSSForSFun__/16(zC) -> zC/1
  __OutputSSForSFun__/17(zD) -> zD/1
  __OutputSSForSFun__/18(zE) -> zE/1
  __OutputSSForSFun__/19(zF) -> zF/1
  __OutputSSForSFun__/20(FA) -> FA/1
  __OutputSSForSFun__/21(FB) -> FB/1
  __OutputSSForSFun__/22(FC) -> FC/1
  __OutputSSForSFun__/23(VA) -> VA/1
  __OutputSSForSFun__/24(VB) -> VB/1
  __OutputSSForSFun__/25(VC) -> VC/1

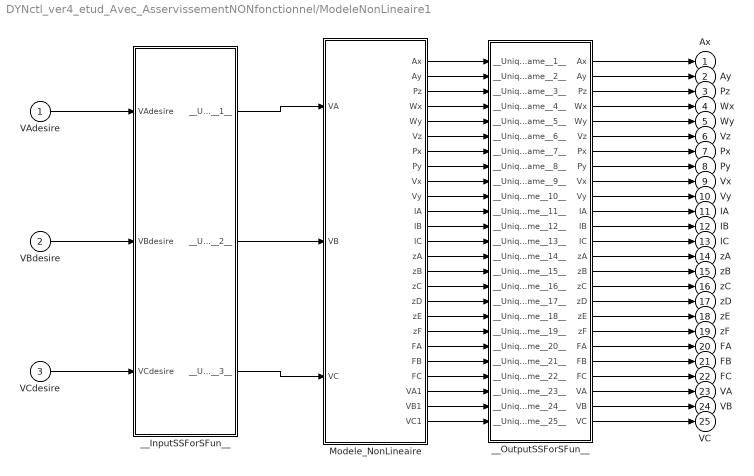
== system DYNctl_ver4_etud_Avec_AsservissementNONfonctionnel/ModeleNonLineaire1 ==
  VAdesire : Inport
  VBdesire : Inport  Port=2
  VCdesire : Inport  Port=3
  Modele_NonLineaire : Subsystem
  __InputSSForSFun__ : Subsystem
  __OutputSSForSFun__ : Subsystem
  Ax : Outport
  Ay : Outport  Port=2
  Pz : Outport  Port=3
  Wx : Outport  Port=4
  Wy : Outport  Port=5
  Vz : Outport  Port=6
  Px : Outport  Port=7
  Py : Outport  Port=8
  Vx : Outport  Port=9
  Vy : Outport  Port=10
  IA : Outport  Port=11
  IB : Outport  Port=12
  IC : Outport  Port=13
  zA : Outport  Port=14
  zB : Outport  Port=15
  zC : Outport  Port=16
  zD : Outport  Port=17
  zE : Outport  Port=18
  zF : Outport  Port=19
  FA : Outport  Port=20
  FB : Outport  Port=21
  FC : Outport  Port=22
  VA : Outport  Port=23
  VB : Outport  Port=24
  VC : Outport  Port=25
  wires:
  VAdesire/1 -> __InputSSForSFun__/1(VAdesire)
  VBdesire/1 -> __InputSSForSFun__/2(VBdesire)
  VCdesire/1 -> __InputSSForSFun__/3(VCdesire)
  __InputSSForSFun__/1(__UniqueOutportName__1__) -> Modele_NonLineaire/1(VA)
  __InputSSForSFun__/2(__UniqueOutportName__2__) -> Modele_NonLineaire/2(VB)
  __InputSSForSFun__/3(__UniqueOutportName__3__) -> Modele_NonLineaire/3(VC)
  Modele_NonLineaire/1(Ax) -> __OutputSSForSFun__/1(__UniqueInportName__1__)
  Modele_NonLineaire/2(Ay) -> __OutputSSForSFun__/2(__UniqueInportName__2__)
  Modele_NonLineaire/3(Pz) -> __OutputSSForSFun__/3(__UniqueInportName__3__)
  Modele_NonLineaire/4(Wx) -> __OutputSSForSFun__/4(__UniqueInportName__4__)
  Modele_NonLineaire/5(Wy) -> __OutputSSForSFun__/5(__UniqueInportName__5__)
  Modele_NonLineaire/6(Vz) -> __OutputSSForSFun__/6(__UniqueInportName__6__)
  Modele_NonLineaire/7(Px) -> __OutputSSForSFun__/7(__UniqueInportName__7__)
  Modele_NonLineaire/8(Py) -> __OutputSSForSFun__/8(__UniqueInportName__8__)
  Modele_NonLineaire/9(Vx) -> __OutputSSForSFun__/9(__UniqueInportName__9__)
  Modele_NonLineaire/10(Vy) -> __OutputSSForSFun__/10(__UniqueInportName__10__)
  Modele_NonLineaire/11(IA) -> __OutputSSForSFun__/11(__UniqueInportName__11__)
  Modele_NonLineaire/12(IB) -> __OutputSSForSFun__/12(__UniqueInportName__12__)
  Modele_NonLineaire/13(IC) -> __OutputSSForSFun__/13(__UniqueInportName__13__)
  Modele_NonLineaire/14(zA) -> __OutputSSForSFun__/14(__UniqueInportName__14__)
  Modele_NonLineaire/15(zB) -> __OutputSSForSFun__/15(__UniqueInportName__15__)
  Modele_NonLineaire/16(zC) -> __OutputSSForSFun__/16(__UniqueInportName__16__)
  Modele_NonLineaire/17(zD) -> __OutputSSForSFun__/17(__UniqueInportName__17__)
  Modele_NonLineaire/18(zE) -> __OutputSSForSFun__/18(__UniqueInportName__18__)
  Modele_NonLineaire/19(zF) -> __OutputSSForSFun__/19(__UniqueInportName__19__)
  Modele_NonLineaire/20(FA) -> __OutputSSForSFun__/20(__UniqueInportName__20__)
  Modele_NonLineaire/21(FB) -> __OutputSSForSFun__/21(__UniqueInportName__21__)
  Modele_NonLineaire/22(FC) -> __OutputSSForSFun__/22(__UniqueInportName__22__)
  Modele_NonLineaire/23(VA1) -> __OutputSSForSFun__/23(__UniqueInportName__23__)
  Modele_NonLineaire/24(VB1) -> __OutputSSForSFun__/24(__UniqueInportName__24__)
  Modele_NonLineaire/25(VC1) -> __OutputSSForSFun__/25(__UniqueInportName__25__)
  __OutputSSForSFun__/1(Ax) -> Ax/1
  __OutputSSForSFun__/2(Ay) -> Ay/1
  __OutputSSForSFun__/3(Pz) -> Pz/1
  __OutputSSForSFun__/4(Wx) -> Wx/1
  __OutputSSForSFun__/5(Wy) -> Wy/1
  __OutputSSForSFun__/6(Vz) -> Vz/1
  __OutputSSForSFun__/7(Px) -> Px/1
  __OutputSSForSFun__/8(Py) -> Py/1
  __OutputSSForSFun__/9(Vx) -> Vx/1
  __OutputSSForSFun__/10(Vy) -> Vy/1
  __OutputSSForSFun__/11(IA) -> IA/1
  __OutputSSForSFun__/12(IB) -> IB/1
  __OutputSSForSFun__/13(IC) -> IC/1
  __OutputSSForSFun__/14(zA) -> zA/1
  __OutputSSForSFun__/15(zB) -> zB/1
  __OutputSSForSFun__/16(zC) -> zC/1
  __OutputSSForSFun__/17(zD) -> zD/1
  __OutputSSForSFun__/18(zE) -> zE/1
  __OutputSSForSFun__/19(zF) -> zF/1
  __OutputSSForSFun__/20(FA) -> FA/1
  __OutputSSForSFun__/21(FB) -> FB/1
  __OutputSSForSFun__/22(FC) -> FC/1
  __OutputSSForSFun__/23(VA) -> VA/1
  __OutputSSForSFun__/24(VB) -> VB/1
  __OutputSSForSFun__/25(VC) -> VC/1

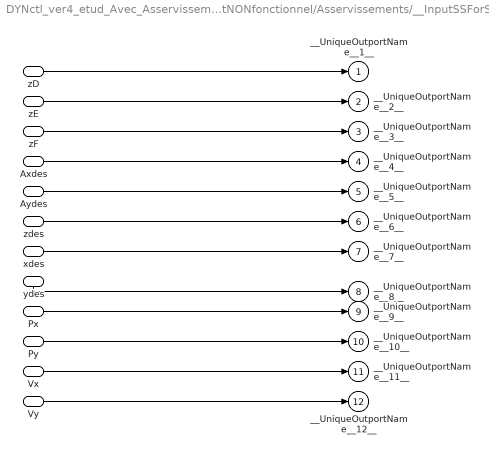
== system DYNctl_ver4_etud_Avec_AsservissementNONfonctionnel/Asservissements/__InputSSForSFun__ ==
  zD : Inport
  zE : Inport  Port=2
  zF : Inport  Port=3
  Axdes : Inport  Port=4
  Aydes : Inport  Port=5
  zdes : Inport  Port=6
  xdes : Inport  Port=7
  ydes : Inport  Port=8
  Px : Inport  Port=9
  Py : Inport  Port=10
  Vx : Inport  Port=11
  Vy : Inport  Port=12
  __UniqueOutportName__1__ : Outport
  __UniqueOutportName__2__ : Outport  Port=2
  __UniqueOutportName__3__ : Outport  Port=3
  __UniqueOutportName__4__ : Outport  Port=4
  __UniqueOutportName__5__ : Outport  Port=5
  __UniqueOutportName__6__ : Outport  Port=6
  __UniqueOutportName__7__ : Outport  Port=7
  __UniqueOutportName__8__ : Outport  Port=8
  __UniqueOutportName__9__ : Outport  Port=9
  __UniqueOutportName__10__ : Outport  Port=10
  __UniqueOutportName__11__ : Outport  Port=11
  __UniqueOutportName__12__ : Outport  Port=12
  wires:
  zD/1 -> __UniqueOutportName__1__/1
  zE/1 -> __UniqueOutportName__2__/1
  zF/1 -> __UniqueOutportName__3__/1
  Axdes/1 -> __UniqueOutportName__4__/1
  Aydes/1 -> __UniqueOutportName__5__/1
  zdes/1 -> __UniqueOutportName__6__/1
  xdes/1 -> __UniqueOutportName__7__/1
  ydes/1 -> __UniqueOutportName__8__/1
  Px/1 -> __UniqueOutportName__9__/1
  Py/1 -> __UniqueOutportName__10__/1
  Vx/1 -> __UniqueOutportName__11__/1
  Vy/1 -> __UniqueOutportName__12__/1

== system DYNctl_ver4_etud_Avec_AsservissementNONfonctionnel/Asservissements/__OutputSSForSFun__ ==
  __UniqueInportName__1__ : Inport
  __UniqueInportName__2__ : Inport  Port=2
  __UniqueInportName__3__ : Inport  Port=3
  __UniqueInportName__4__ : Inport  Port=4
  __UniqueInportName__5__ : Inport  Port=5
  VAcalcule : Outport
  VBcalcule : Outport  Port=2
  VCcalcule : Outport  Port=3
  Axcalcule : Outport  Port=4
  Aycalcule : Outport  Port=5
  wires:
  __UniqueInportName__1__/1 -> VAcalcule/1
  __UniqueInportName__2__/1 -> VBcalcule/1
  __UniqueInportName__3__/1 -> VCcalcule/1
  __UniqueInportName__4__/1 -> Axcalcule/1  "Ax_des"
  __UniqueInportName__5__/1 -> Aycalcule/1  "Ay_des"

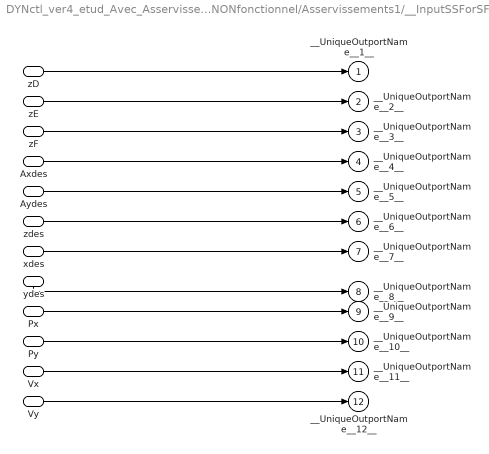
== system DYNctl_ver4_etud_Avec_AsservissementNONfonctionnel/Asservissements1/__InputSSForSFun__ ==
  zD : Inport
  zE : Inport  Port=2
  zF : Inport  Port=3
  Axdes : Inport  Port=4
  Aydes : Inport  Port=5
  zdes : Inport  Port=6
  xdes : Inport  Port=7
  ydes : Inport  Port=8
  Px : Inport  Port=9
  Py : Inport  Port=10
  Vx : Inport  Port=11
  Vy : Inport  Port=12
  __UniqueOutportName__1__ : Outport
  __UniqueOutportName__2__ : Outport  Port=2
  __UniqueOutportName__3__ : Outport  Port=3
  __UniqueOutportName__4__ : Outport  Port=4
  __UniqueOutportName__5__ : Outport  Port=5
  __UniqueOutportName__6__ : Outport  Port=6
  __UniqueOutportName__7__ : Outport  Port=7
  __UniqueOutportName__8__ : Outport  Port=8
  __UniqueOutportName__9__ : Outport  Port=9
  __UniqueOutportName__10__ : Outport  Port=10
  __UniqueOutportName__11__ : Outport  Port=11
  __UniqueOutportName__12__ : Outport  Port=12
  wires:
  zD/1 -> __UniqueOutportName__1__/1
  zE/1 -> __UniqueOutportName__2__/1
  zF/1 -> __UniqueOutportName__3__/1
  Axdes/1 -> __UniqueOutportName__4__/1
  Aydes/1 -> __UniqueOutportName__5__/1
  zdes/1 -> __UniqueOutportName__6__/1
  xdes/1 -> __UniqueOutportName__7__/1
  ydes/1 -> __UniqueOutportName__8__/1
  Px/1 -> __UniqueOutportName__9__/1
  Py/1 -> __UniqueOutportName__10__/1
  Vx/1 -> __UniqueOutportName__11__/1
  Vy/1 -> __UniqueOutportName__12__/1

== system DYNctl_ver4_etud_Avec_AsservissementNONfonctionnel/Asservissements1/__OutputSSForSFun__ ==
  __UniqueInportName__1__ : Inport
  __UniqueInportName__2__ : Inport  Port=2
  __UniqueInportName__3__ : Inport  Port=3
  __UniqueInportName__4__ : Inport  Port=4
  __UniqueInportName__5__ : Inport  Port=5
  VAcalcule : Outport
  VBcalcule : Outport  Port=2
  VCcalcule : Outport  Port=3
  Axcalcule : Outport  Port=4
  Aycalcule : Outport  Port=5
  wires:
  __UniqueInportName__1__/1 -> VAcalcule/1
  __UniqueInportName__2__/1 -> VBcalcule/1
  __UniqueInportName__3__/1 -> VCcalcule/1
  __UniqueInportName__4__/1 -> Axcalcule/1  "Ax_des"
  __UniqueInportName__5__/1 -> Aycalcule/1  "Ay_des"

== system DYNctl_ver4_etud_Avec_AsservissementNONfonctionnel/Asservissements2/Position sphere X2 ==
  xdes : Inport
  Px : Inport  Port=2
  Vx : Inport  Port=3
  Gain : Gain  Gain=Kp_pos_sph
  Gain1 : Gain  Gain=Kv_pos_sph
  Sum : Sum  Inputs=|+-
  Sum1 : Sum  Inputs=|+-
  Axdes : Outport
  wires:
  Gain/1 -> Sum1/1
  xdes/1 -> Sum/1
  Vx/1 -> Gain1/1
  Px/1 -> Sum/2
  Sum1/1 -> Axdes/1
  Gain1/1 -> Sum1/2
  Sum/1 -> Gain/1

== system DYNctl_ver4_etud_Avec_AsservissementNONfonctionnel/Asservissements2/Position sphere X3 ==
  ydes : Inport
  Py : Inport  Port=2
  Vy : Inport  Port=3
  Gain : Gain  Gain=-Kp_pos_sph
  Gain1 : Gain  Gain=-Kv_pos_sph
  Sum : Sum  Inputs=|+-
  Sum1 : Sum  Inputs=|+-
  Aydes : Outport
  wires:
  Gain/1 -> Sum1/1
  ydes/1 -> Sum/1
  Gain1/1 -> Sum1/2
  Vy/1 -> Gain1/1
  Py/1 -> Sum/2
  Sum1/1 -> Aydes/1
  Sum/1 -> Gain/1
